simulink model "sys_ev"  (R2018b)
settings: Solver=FixedStepAuto  StartTime=0.0  StopTime=24  FixedStep=1  RelTol=1e-3
values from neighbouring files (symbols this model uses):
  c_std = 1 / Cc    (= 0.232558139535)    [sys_evolution.m]
  Cc = cc * mc    (= 4.3)    [sys_evolution.m]
  Cf = cf * mf    (= 1.3)    [sys_evolution.m]
  f_std = 1 / Cf    (= 0.769230769231)    [sys_evolution.m]
  kaf = k_bar_af * sf    (= 7.32)    [sys_evolution.m]
  kfc = k_bar_fc * sc    (= 9.5)    [sys_evolution.m]
  sampling_time = 1    [sys_evolution.m]
settings Model: Creator=Nico  LastModifiedBy=Nico

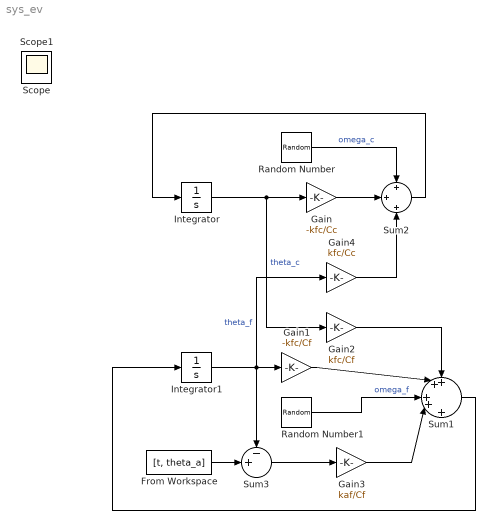
== system sys_ev ==
  From Workspace : FromWorkspace  VariableName=[t, theta_a]  SampleTime=0
  Gain : Gain  Gain=-kfc/Cc
  Gain1 : Gain  Gain=-kfc/Cf
  Gain2 : Gain  Gain=kfc/Cf
  Gain3 : Gain  Gain=kaf/Cf
  Gain4 : Gain  Gain=kfc/Cc
  Integrator : Integrator  InitialCondition=293
  Integrator1 : Integrator  InitialCondition=291
  Random Number : RandomNumber  Variance=c_std^2  SampleTime=sampling_time
  Random Number1 : RandomNumber  Variance=f_std^2  SampleTime=sampling_time
  Sum1 : Sum  Inputs=++|++|+
  Sum2 : Sum  Inputs=+|+|+
  Sum3 : Sum  Inputs=-+|
  Scope : Scope
  Scope1 : Scope
  wires:
  Integrator/1 -> Gain2/1, Gain/1  "theta_c"
  Integrator1/1 -> Gain1/1, Sum3/1, Gain4/1  "theta_f"
  Gain/1 -> Sum2/2
  Random Number/1 -> Sum2/1  "omega_c"
  Sum2/1 -> Integrator/1
  Gain1/1 -> Sum1/2
  Gain2/1 -> Sum1/1
  Sum3/1 -> Gain3/1
  Gain3/1 -> Sum1/4
  Random Number1/1 -> Sum1/3  "omega_f"
  Sum1/1 -> Integrator1/1
  Gain4/1 -> Sum2/3
  From Workspace/1 -> Sum3/2
